simulink model "ANPC_BTB_precharge"  (Simulink 7.3)
settings: Solver=FixedStepDiscrete  StartTime=0.0  StopTime=5  FixedStep=10e-6  RelTol=1e-3
undefined symbols (not defined in the file or in its folder): C, Cd, Cf, Lg
libraries: powerlib x112, simulink x1
settings Model: Creator=wangkui02  LastModifiedBy=wangkui

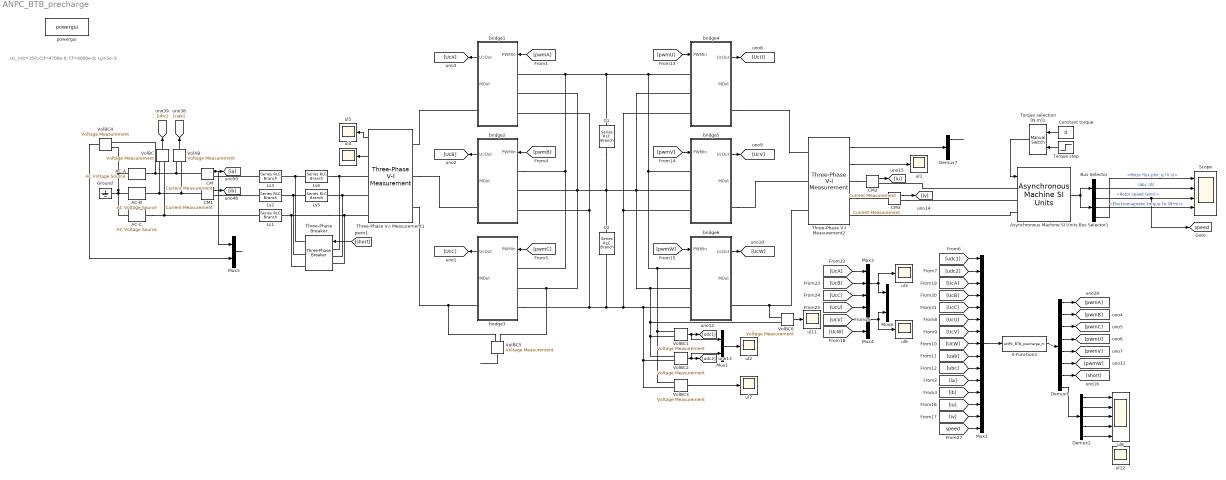
== system ANPC_BTB_precharge ==
  note: Uc_init=150;
      | Cd=4700e-6;
      | Cf=6600e-6;
      | Lg=5e-3;
  AC-A : powerlib/Electrical Sources/AC Voltage Source  DialogController=POWERSYS.PowerSysDialog  SystemSampleTime=-1  Amplitude=311  Phase=0  Frequency=50  SampleTime=0  Measurements=None
  AC-B : powerlib/Electrical Sources/AC Voltage Source  DialogController=POWERSYS.PowerSysDialog  SystemSampleTime=-1  Amplitude=311  Phase=-120  Frequency=50  SampleTime=0  Measurements=None
  AC-C : powerlib/Electrical Sources/AC Voltage Source  DialogController=POWERSYS.PowerSysDialog  SystemSampleTime=-1  Amplitude=311  Phase=120  Frequency=50  SampleTime=0  Measurements=None
  Asynchronous Machine SI Units : powerlib/Machines/Asynchronous Machine SI Units  DialogController=POWERSYS.PowerSysDialog  SystemSampleTime=-1  PresetModel=No  MechanicalLoad=Torque Tm  ShowDetailedParameters=on  RotorType=Squirrel-cage  ReferenceFrame=Stationary  NominalParameters=[2200 380 50]  Stator=[2.74 0.0138]  Rotor=[2.54 0.0138]  Lm=0.299  Mechanical=[0.0131 0.002985 2]  PolePairs=2  InitialConditions="[ 1,0   0,0,0   0,0,0 ]"  Units=SI  LoadFlowParameters=0  SimulateSaturation=off  Saturation=[14.03593122, 27.81365428, 53.79336849, 72.68890987, 97.98006896, 148.6815601, 215.7428561, 302.9841135, 428.7778367 ; 230, 322, 414, 460, 506, 552, 598, 644, 690]  TsPowergui=0  TsBlock=-1  IterativeModel=Forward Euler
  Bus Selector : BusSelector  OutputSignals=Stator measurements.Stator current is_a (A),Stator measurements.Stator current is_b (A),Stator measurements.Stator current is_c (A)  OutputAsBus=on
  Bus Selector1 : BusSelector  OutputSignals=Mechanical.Rotor speed (wm),Mechanical.Electromagnetic torque Te (N*m),Rotor measurements.Rotor flux phir_q (V s)
  C1 : powerlib/Elements/Series RLC Branch  DialogController=POWERSYS.PowerSysDialog  PhysicalDomain=powersysdomain  SubClassName=unknown  LeftPortType=p1  RightPortType=p1  LConnTagsString=__new0  RConnTagsString=__new0  BranchType=C  Resistance=1  Inductance=1e-3  SetiL0=off  InitialCurrent=0  Capacitance=Cd  Setx0=on  InitialVoltage=0  Measurements=None
  C2 : powerlib/Elements/Series RLC Branch  DialogController=POWERSYS.PowerSysDialog  PhysicalDomain=powersysdomain  SubClassName=unknown  LeftPortType=p1  RightPortType=p1  LConnTagsString=__new0  RConnTagsString=__new0  BranchType=C  Resistance=1  Inductance=1e-3  SetiL0=off  InitialCurrent=0  Capacitance=Cd  Setx0=on  InitialVoltage=0  Measurements=None
  CM{,1..3} (4 alike) : powerlib/Measurements/Current Measurement  DialogController=POWERSYS.PowerSysDialog  SystemSampleTime=-1  PhasorSimulation=off  OutputType=Complex  PSBequivalent=0
  Constant torque : Constant  Value=0  OutDataType=sfix(16)  OutScaling=2^0
  Demux1 : Demux  Outputs=[12 12 12 12 12 12 1 5]
  Demux2 : Demux  Outputs=5
  Demux7 : Demux  Outputs=3
  Ground : powerlib/Elements/Ground  DialogController=POWERSYS.PowerSysDialog  PhysicalDomain=powersysdomain  SubClassName=unknown  LeftPortType=p1  RightPortType=p1  LConnTagsString=a
  Ls1 : powerlib/Elements/Series RLC Branch  DialogController=POWERSYS.PowerSysDialog  PhysicalDomain=powersysdomain  SubClassName=unknown  LeftPortType=p1  RightPortType=p1  LConnTagsString=__new0  RConnTagsString=__new0  BranchType=L  Resistance=1  Inductance=Lg  SetiL0=off  InitialCurrent=0  Capacitance=C  Setx0=on  InitialVoltage=Uc  Measurements=Branch voltage and current
  Ls2 : powerlib/Elements/Series RLC Branch  DialogController=POWERSYS.PowerSysDialog  PhysicalDomain=powersysdomain  SubClassName=unknown  LeftPortType=p1  RightPortType=p1  LConnTagsString=__new0  RConnTagsString=__new0  BranchType=L  Resistance=1  Inductance=Lg  SetiL0=off  InitialCurrent=0  Capacitance=C  Setx0=on  InitialVoltage=Uc  Measurements=Branch voltage and current
  Ls3 : powerlib/Elements/Series RLC Branch  DialogController=POWERSYS.PowerSysDialog  PhysicalDomain=powersysdomain  SubClassName=unknown  LeftPortType=p1  RightPortType=p1  LConnTagsString=__new0  RConnTagsString=__new0  BranchType=L  Resistance=1  Inductance=Lg  SetiL0=off  InitialCurrent=0  Capacitance=C  Setx0=on  InitialVoltage=Uc  Measurements=Branch voltage and current
  Ls5 : powerlib/Elements/Series RLC Branch  DialogController=POWERSYS.PowerSysDialog  PhysicalDomain=powersysdomain  SubClassName=unknown  LeftPortType=p1  RightPortType=p1  LConnTagsString=__new0  RConnTagsString=__new0  BranchType=R  Resistance=20  Inductance=Lg  SetiL0=off  InitialCurrent=0  Capacitance=C  Setx0=on  InitialVoltage=Uc  Measurements=Branch voltage and current
  Ls6 : powerlib/Elements/Series RLC Branch  DialogController=POWERSYS.PowerSysDialog  PhysicalDomain=powersysdomain  SubClassName=unknown  LeftPortType=p1  RightPortType=p1  LConnTagsString=__new0  RConnTagsString=__new0  BranchType=R  Resistance=20  Inductance=Lg  SetiL0=off  InitialCurrent=0  Capacitance=C  Setx0=on  InitialVoltage=Uc  Measurements=Branch voltage and current
  Mux1 : Mux  Inputs=2
  Mux2 : Mux  Inputs=15
  Mux3 : Mux  Inputs=3
  Mux4 : Mux  Inputs=3
  Mux5 : Mux  Inputs=2
  Mux6 : Mux  Inputs=2
  S-Function2 : S-Function  FunctionName=ANPC_BTB_precharge_m  EnableBusSupport=off
  Scope : Scope  NumInputPorts=4
      settings: YMin=-1~-12.5~-10~-2.5  YMax=1~12.5~110~22.5  SaveName=ScopeData9  Decimation=20  SampleTime=5e-6
  Three-Phase V-I Measurement1 : powerlib/Measurements/Three-Phase V-I Measurement  DialogController=POWERSYS.PowerSysDialog  SystemSampleTime=-1  VoltageMeasurement=phase-to-phase  SetLabelV=off  LabelV=Vabc  Vpu=off  CurrentMeasurement=yes  SetLabelI=off  LabelI=Iabc  Ipu=off  Pbase=100e6  Vbase=500e3  OutputType=Complex  PhasorSimulation=off  PSBequivalent=0
  Three-Phase V-I Measurement2 : powerlib/Measurements/Three-Phase V-I Measurement  DialogController=POWERSYS.PowerSysDialog  SystemSampleTime=-1  VoltageMeasurement=phase-to-phase  SetLabelV=off  LabelV=Vabc  Vpu=off  CurrentMeasurement=yes  SetLabelI=off  LabelI=Iabc  Ipu=off  Pbase=100e6  Vbase=500e3  OutputType=Complex  PhasorSimulation=off  PSBequivalent=0
  Three-Phase Breaker : powerlib/Elements/Three-Phase Breaker  DialogController=POWERSYS.PowerSysDialog  SystemSampleTime=-1  InitialState=open  SwitchA=on  SwitchB=on  SwitchC=on  SwitchTimes="[4/60  10/60]"  External=on  BreakerResistance=0.001  SnubberResistance=1e6  SnubberCapacitance=inf  Measurements=None
  Torque selection (N.m)1 : simulink/Signal Routing/Manual Switch  SystemSampleTime=-1  sw=0  action=0  varsize=off
  Torque step : Step  Time=3.5  After=10  SampleTime=0
  VolAB : powerlib/Measurements/Voltage Measurement  DialogController=POWERSYS.PowerSysDialog  SystemSampleTime=-1  PhasorSimulation=off  OutputType=Complex  PSBequivalent=0
  VolBC{,1..6} (7 alike) : powerlib/Measurements/Voltage Measurement  DialogController=POWERSYS.PowerSysDialog  SystemSampleTime=-1  PhasorSimulation=off  OutputType=Complex  PSBequivalent=0
  bridge1 : Subsystem
  bridge2 : Subsystem
  bridge3 : Subsystem
  bridge4 : Subsystem
  bridge5 : Subsystem
  bridge6 : Subsystem
  powergui : powerlib/powergui  SystemSampleTime=-1  SimulationMode=Discrete  SampleTime=10e-6  frequency=60  SPID=off  DisableSnubberDevices=off  DisableRonSwitches=off  DisableVfSwitches=off  SwTol=0  Interpol=off  frequencyindice=0  echomessages=off  HookPort=off  DisplayEquations=off  FunctionMessages=off  EnableUseOfTLC=off  x0status=blocks  RestoreLinks=warning  Frange=[0:2:500]  Ylog=off  Xlog=on  ShowGrid=off  save=off  variable=ZData  ZoomFFT=on  StartTime=0.0  cycles=1  DisplayStyle=1  fundamental=60  FreqAxis=off  MaxFrequency=1000  frequencyindicesteady=1  RmsSteady=1  display=off  Ts=0  methode=off
  ul{1..7,11..12} (9 alike) : Scope
      ul1 settings: YMin=-4  YMax=6  DataFormat=Structure  MaxDataPoints=100000  Decimation=10
      ul11 settings: YMin=-350  YMax=350  SaveName=ScopeData11  DataFormat=Structure  MaxDataPoints=100000  Decimation=10
      ul12 settings: YMin=-2  YMax=4  SaveName=ScopeData12  DataFormat=Structure  MaxDataPoints=100000  Decimation=10
      ul2 settings: TimeRange=1  YMin=297.5  YMax=302.5  SaveName=ScopeData2  DataFormat=Structure  MaxDataPoints=100000  Decimation=10
      ul3 settings: YMin=149.3  YMax=150.7  DataFormat=Structure  MaxDataPoints=100000  Decimation=10
      ul4 settings: YMin=-11  YMax=11  SaveName=ScopeData3  DataFormat=Structure  MaxDataPoints=100000  Decimation=10
      ul5 settings: YMin=-0.0225  YMax=0.0225  SaveName=ScopeData4  DataFormat=Structure  MaxDataPoints=100000  Decimation=10
      ul6 settings: YMin=0  YMax=160  SaveName=ScopeData5  DataFormat=Structure  MaxDataPoints=100000  Decimation=10
      ul7 settings: YMin=599  YMax=601.4  SaveName=ScopeData6  DataFormat=Structure  MaxDataPoints=100000  Decimation=10
  ul8 : Scope  NumInputPorts=5
      settings: YMin=-15~-5~0~-1.25e-013~-4  YMax=40~30~350~1.25e-013~4  SaveName=ScopeData7  DataFormat=Structure  MaxDataPoints=100000
  tag scope: speed=global
  wires:
  VolAB/1 -> [uab]
  VolBC/1 -> [ubc]
  [pwmB] -> bridge2/1(PWMIn)
  [pwmC] -> bridge3/1(PWMIn)
  CM/1 -> [ia], Mux5/1
  CM1/1 -> [ib]
  [pwmU] -> bridge4/1(PWMIn)
  [pwmV] -> bridge5/1(PWMIn)
  [pwmW] -> bridge6/1(PWMIn)
  bridge4/1(UcOut) -> [UcU]
  bridge5/1(UcOut) -> [UcV]
  bridge6/1(UcOut) -> [UcW]
  [pwmA] -> bridge1/1(PWMIn)
  bridge3/1(UcOut) -> [UcC]
  bridge2/1(UcOut) -> [UcB]
  bridge1/1(UcOut) -> [UcA]
  Three-Phase V-I Measurement2/2 -> ul1/1
  Demux7/1 -> ?
  Three-Phase V-I Measurement2/1 -> Demux7/1
  CM2/1 -> [iu]
  CM3/1 -> [iv]
  VolBC2/1 -> [udc2], Mux1/2
  VolBC1/1 -> [udc1], Mux1/1
  Mux1/1 -> ul2/1
  VolBC3/1 -> ul7/1
  Three-Phase V-I Measurement1/1 -> ul5/1
  Three-Phase V-I Measurement1/2 -> ul4/1
  Mux5/1 -> ?
  VolBC4/1 -> Mux5/2
  Mux2/1 -> S-Function2/1
  S-Function2/1 -> Demux1/1
  Demux1/1 -> [pwmA]
  Demux1/2 -> [pwmB]
  Demux1/3 -> [pwmC]
  [udc1] -> Mux2/1
  [udc2] -> Mux2/2
  [UcA] -> Mux2/3
  [UcB] -> Mux2/4
  [UcC] -> Mux2/5
  [UcU] -> Mux2/6
  [UcV] -> Mux2/7
  [UcW] -> Mux2/8
  [uab] -> Mux2/9
  [ubc] -> Mux2/10
  [ia] -> Mux2/11
  [ib] -> Mux2/12
  [iu] -> Mux2/13
  [iv] -> Mux2/14
  Demux1/4 -> [pwmU]
  Demux1/5 -> [pwmV]
  Demux1/6 -> [pwmW]
  Demux2/3 -> ul8/3
  Demux2/1 -> ul8/1
  Demux2/2 -> ul8/2
  Demux2/4 -> ul8/4
  [speed] -> Mux2/15
  [UcA] -> Mux3/1
  [UcB] -> Mux3/2
  [UcC] -> Mux3/3
  [UcU] -> Mux4/1
  [UcV] -> Mux4/2
  [UcW] -> Mux4/3
  VolBC5/1 -> ?
  VolBC6/1 -> ul11/1
  Mux3/1 -> Mux6/1, ul3/1
  Mux4/1 -> Mux6/2, ul6/1
  Bus Selector1/1 -> Scope/3, [speed]  "<Rotor speed (wm)>"
  Bus Selector/1 -> Scope/2  "Iabc (A)"
  Bus Selector1/2 -> Scope/4  "<Electromagnetic torque Te (N*m)>"
  Asynchronous Machine SI Units/1 -> Bus Selector/1, Bus Selector1/1
  Torque selection (N.m)1/1 -> Asynchronous Machine SI Units/1
  Constant torque/1 -> Torque selection (N.m)1/1
  Torque step/1 -> Torque selection (N.m)1/2
  Bus Selector1/3 -> Scope/1  "<Rotor flux phir_q (V s)>"
  [short] -> Three-Phase Breaker/1
  Demux1/8 -> Demux2/1
  Demux1/7 -> [short]
  Demux2/5 -> ul8/5
  connections:
  AC-A/RConn1 -- VolAB/LConn1 -- CM/LConn1 -- VolBC4/LConn1
  AC-C/RConn1 -- Ls1/LConn1 -- VolBC/LConn2
  Ground/LConn1 -- AC-B/LConn1 -- AC-C/LConn1 -- AC-A/LConn1 -- VolBC4/LConn2
  Three-Phase V-I Measurement1/LConn1 -- bridge1/RConn1
  Three-Phase V-I Measurement1/LConn2 -- bridge2/RConn1
  Three-Phase V-I Measurement1/LConn3 -- bridge3/RConn1 -- VolBC5/LConn1
  CM1/RConn1 -- Ls2/LConn1
  Ls3/LConn1 -- CM/RConn1
  bridge6/LConn1 -- bridge3/LConn1 -- bridge2/LConn1 -- bridge1/LConn1 -- C1/LConn1 -- bridge4/LConn1 -- bridge5/LConn1 -- VolBC1/LConn1 -- VolBC3/LConn1
  bridge6/LConn3 -- bridge3/LConn3 -- bridge1/LConn3 -- bridge2/LConn3 -- C2/RConn1 -- bridge4/LConn3 -- bridge5/LConn3 -- VolBC2/LConn2 -- VolBC3/LConn2
  bridge4/RConn1 -- Three-Phase V-I Measurement2/LConn1
  bridge5/RConn1 -- Three-Phase V-I Measurement2/LConn2
  bridge6/RConn1 -- Three-Phase V-I Measurement2/LConn3 -- VolBC6/LConn1
  VolBC/LConn1 -- AC-B/RConn1 -- CM1/LConn1 -- VolAB/LConn2
  Three-Phase V-I Measurement2/RConn1 -- CM2/LConn1
  Three-Phase V-I Measurement2/RConn2 -- CM3/LConn1
  VolBC2/LConn1 -- VolBC1/LConn2 -- C2/LConn1 -- bridge2/LConn2 -- bridge1/LConn2 -- bridge3/LConn2 -- VolBC5/LConn2 -- C1/RConn1 -- bridge4/LConn2 -- bridge5/LConn2 -- bridge6/LConn2 -- VolBC6/LConn2
  CM3/RConn1 -- Asynchronous Machine SI Units/LConn2
  Three-Phase V-I Measurement2/RConn3 -- Asynchronous Machine SI Units/LConn3
  Asynchronous Machine SI Units/LConn1 -- CM2/RConn1
  Ls6/LConn1 -- Ls3/RConn1 -- Three-Phase Breaker/RConn1
  Ls5/LConn1 -- Ls2/RConn1 -- Three-Phase Breaker/RConn2
  Ls6/RConn1 -- Three-Phase V-I Measurement1/RConn1 -- Three-Phase Breaker/LConn1
  Ls5/RConn1 -- Three-Phase V-I Measurement1/RConn2 -- Three-Phase Breaker/LConn2
  Ls1/RConn1 -- Three-Phase Breaker/RConn3 -- Three-Phase V-I Measurement1/RConn3 -- Three-Phase Breaker/LConn3

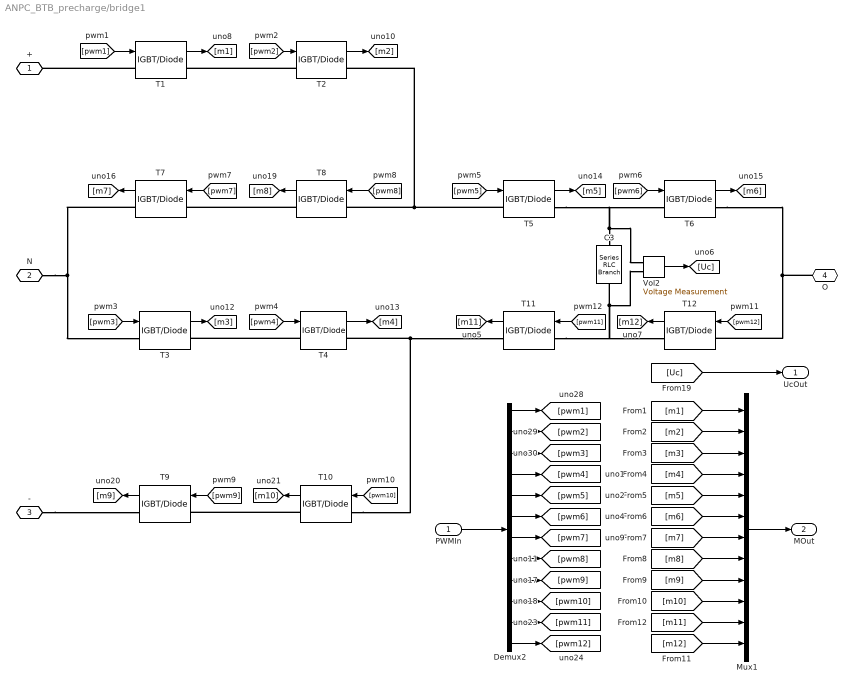
== system ANPC_BTB_precharge/bridge1 ==
  PWMIn : Inport
  C3 : powerlib/Elements/Series RLC Branch  DialogController=POWERSYS.PowerSysDialog  PhysicalDomain=powersysdomain  SubClassName=unknown  LeftPortType=p1  RightPortType=p1  LConnTagsString=__new0  RConnTagsString=__new0  BranchType=C  Resistance=1  Inductance=1e-3  SetiL0=off  InitialCurrent=0  Capacitance=Cf  Setx0=on  InitialVoltage=0  Measurements=None
  Demux2 : Demux  Outputs=12
  Mux1 : Mux  Inputs=12
  T{1..12} (12 alike) : powerlib/Power Electronics/IGBT//Diode  DialogController=POWERSYS.PowerSysDialog  SystemSampleTime=-1  Ron=1e-3  Rs=1e5  Cs=inf  Measurements=on
  Vol2 : powerlib/Measurements/Voltage Measurement  DialogController=POWERSYS.PowerSysDialog  SystemSampleTime=-1  PhasorSimulation=off  OutputType=Complex  PSBequivalent=0
  + : PMIOPort  Port=1  Side=Left
  N : PMIOPort  Port=2  Side=Left
  - : PMIOPort  Port=3  Side=Left
  O : PMIOPort  Port=4  Side=Right
  UcOut : Outport  OutDataType=fixdt(1, 16)  OutScaling=2^0
  MOut : Outport  Port=2  OutDataType=fixdt(1, 16)  OutScaling=2^0
  wires:
  T1/1 -> [m1]
  [pwm10] -> T10/1
  T10/1 -> [m10]
  [pwm3] -> T3/1
  T3/1 -> [m3]
  [pwm4] -> T4/1
  T4/1 -> [m4]
  [pwm5] -> T5/1
  T5/1 -> [m5]
  [pwm2] -> T2/1
  T2/1 -> [m2]
  [pwm6] -> T6/1
  T6/1 -> [m6]
  [pwm7] -> T7/1
  [pwm8] -> T8/1
  T8/1 -> [m8]
  [pwm9] -> T9/1
  T9/1 -> [m9]
  PWMIn/1 -> Demux2/1
  Demux2/1 -> [pwm1]
  Demux2/2 -> [pwm2]
  Demux2/3 -> [pwm3]
  Demux2/4 -> [pwm4]
  Demux2/5 -> [pwm5]
  Demux2/6 -> [pwm6]
  Demux2/7 -> [pwm7]
  Demux2/8 -> [pwm8]
  Demux2/9 -> [pwm9]
  Demux2/10 -> [pwm10]
  [pwm1] -> T1/1
  T7/1 -> [m7]
  [m1] -> Mux1/1
  [m2] -> Mux1/2
  [m3] -> Mux1/3
  [m4] -> Mux1/4
  [m5] -> Mux1/5
  [m6] -> Mux1/6
  [m7] -> Mux1/7
  [m8] -> Mux1/8
  [m9] -> Mux1/9
  [m10] -> Mux1/10
  Mux1/1 -> MOut/1
  [pwm12] -> T12/1
  T12/1 -> [m12]
  [pwm11] -> T11/1
  T11/1 -> [m11]
  Vol2/1 -> [Uc]
  Demux2/11 -> [pwm11]
  Demux2/12 -> [pwm12]
  [m11] -> Mux1/11
  [m12] -> Mux1/12
  [Uc] -> UcOut/1
  connections:
  T2/LConn1 -- T1/RConn1
  T8/RConn1 -- T7/LConn1
  T1/LConn1 -- +/RConn1
  T7/RConn1 -- T3/LConn1 -- N/RConn1
  -/RConn1 -- T9/RConn1
  T4/LConn1 -- T3/RConn1
  T10/RConn1 -- T9/LConn1
  T11/LConn1 -- T12/RConn1 -- C3/RConn1 -- Vol2/LConn2
  T5/RConn1 -- T6/LConn1 -- C3/LConn1 -- Vol2/LConn1
  T5/LConn1 -- T2/RConn1 -- T8/LConn1
  T10/LConn1 -- T4/RConn1 -- T11/RConn1
  T6/RConn1 -- T12/LConn1 -- O/RConn1

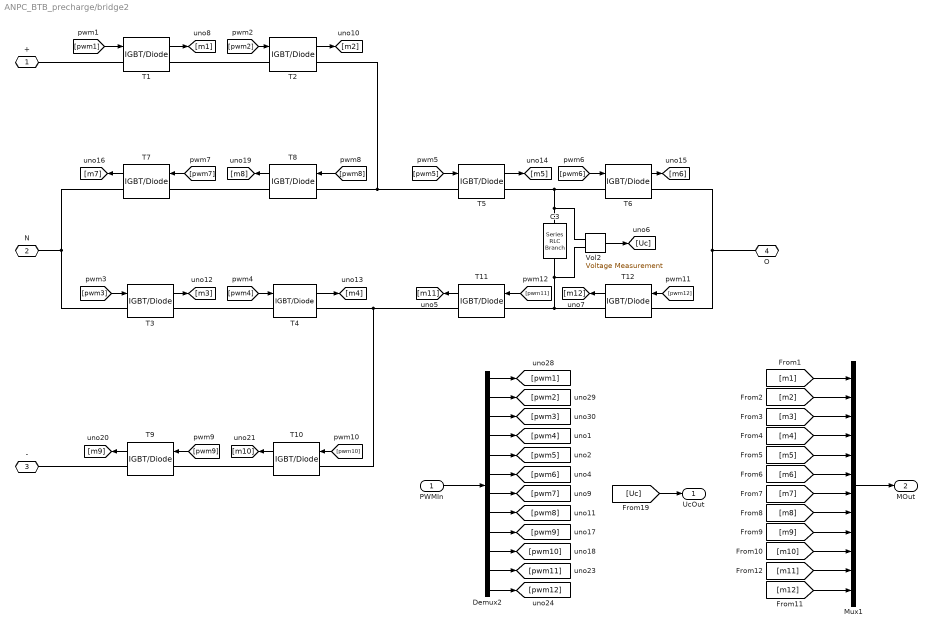
== system ANPC_BTB_precharge/bridge2 ==
  PWMIn : Inport
  C3 : powerlib/Elements/Series RLC Branch  DialogController=POWERSYS.PowerSysDialog  PhysicalDomain=powersysdomain  SubClassName=unknown  LeftPortType=p1  RightPortType=p1  LConnTagsString=__new0  RConnTagsString=__new0  BranchType=C  Resistance=1  Inductance=1e-3  SetiL0=off  InitialCurrent=0  Capacitance=Cf  Setx0=on  InitialVoltage=0  Measurements=None
  Demux2 : Demux  Outputs=12
  Mux1 : Mux  Inputs=12
  T{1..12} (12 alike) : powerlib/Power Electronics/IGBT//Diode  DialogController=POWERSYS.PowerSysDialog  SystemSampleTime=-1  Ron=1e-3  Rs=1e5  Cs=inf  Measurements=on
  Vol2 : powerlib/Measurements/Voltage Measurement  DialogController=POWERSYS.PowerSysDialog  SystemSampleTime=-1  PhasorSimulation=off  OutputType=Complex  PSBequivalent=0
  + : PMIOPort  Port=1  Side=Left
  N : PMIOPort  Port=2  Side=Left
  - : PMIOPort  Port=3  Side=Left
  O : PMIOPort  Port=4  Side=Right
  UcOut : Outport  OutDataType=fixdt(1, 16)  OutScaling=2^0
  MOut : Outport  Port=2  OutDataType=fixdt(1, 16)  OutScaling=2^0
  wires:
  T1/1 -> [m1]
  [pwm10] -> T10/1
  T10/1 -> [m10]
  [pwm3] -> T3/1
  T3/1 -> [m3]
  [pwm4] -> T4/1
  T4/1 -> [m4]
  [pwm5] -> T5/1
  T5/1 -> [m5]
  [pwm2] -> T2/1
  T2/1 -> [m2]
  [pwm6] -> T6/1
  T6/1 -> [m6]
  [pwm7] -> T7/1
  [pwm8] -> T8/1
  T8/1 -> [m8]
  [pwm9] -> T9/1
  T9/1 -> [m9]
  PWMIn/1 -> Demux2/1
  Demux2/1 -> [pwm1]
  Demux2/2 -> [pwm2]
  Demux2/3 -> [pwm3]
  Demux2/4 -> [pwm4]
  Demux2/5 -> [pwm5]
  Demux2/6 -> [pwm6]
  Demux2/7 -> [pwm7]
  Demux2/8 -> [pwm8]
  Demux2/9 -> [pwm9]
  Demux2/10 -> [pwm10]
  [pwm1] -> T1/1
  T7/1 -> [m7]
  [m1] -> Mux1/1
  [m2] -> Mux1/2
  [m3] -> Mux1/3
  [m4] -> Mux1/4
  [m5] -> Mux1/5
  [m6] -> Mux1/6
  [m7] -> Mux1/7
  [m8] -> Mux1/8
  [m9] -> Mux1/9
  [m10] -> Mux1/10
  Mux1/1 -> MOut/1
  [pwm12] -> T12/1
  T12/1 -> [m12]
  [pwm11] -> T11/1
  T11/1 -> [m11]
  Vol2/1 -> [Uc]
  Demux2/11 -> [pwm11]
  Demux2/12 -> [pwm12]
  [m11] -> Mux1/11
  [m12] -> Mux1/12
  [Uc] -> UcOut/1
  connections:
  T2/LConn1 -- T1/RConn1
  T8/RConn1 -- T7/LConn1
  T1/LConn1 -- +/RConn1
  T7/RConn1 -- T3/LConn1 -- N/RConn1
  -/RConn1 -- T9/RConn1
  T4/LConn1 -- T3/RConn1
  T10/RConn1 -- T9/LConn1
  T11/LConn1 -- T12/RConn1 -- C3/RConn1 -- Vol2/LConn2
  T5/RConn1 -- T6/LConn1 -- C3/LConn1 -- Vol2/LConn1
  T5/LConn1 -- T2/RConn1 -- T8/LConn1
  T10/LConn1 -- T4/RConn1 -- T11/RConn1
  T6/RConn1 -- T12/LConn1 -- O/RConn1

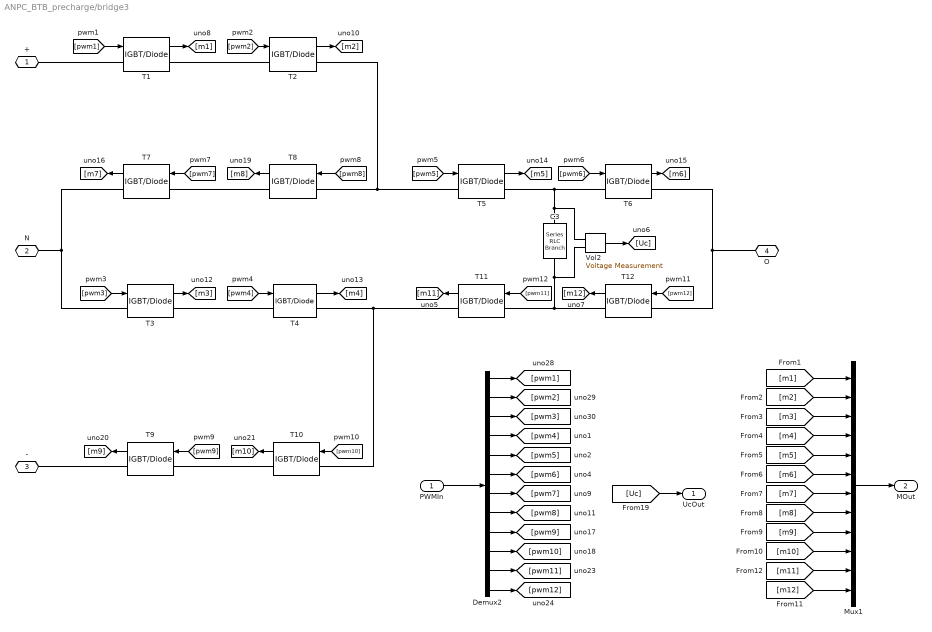
== system ANPC_BTB_precharge/bridge3 ==
  PWMIn : Inport
  C3 : powerlib/Elements/Series RLC Branch  DialogController=POWERSYS.PowerSysDialog  PhysicalDomain=powersysdomain  SubClassName=unknown  LeftPortType=p1  RightPortType=p1  LConnTagsString=__new0  RConnTagsString=__new0  BranchType=C  Resistance=1  Inductance=1e-3  SetiL0=off  InitialCurrent=0  Capacitance=Cf  Setx0=on  InitialVoltage=0  Measurements=None
  Demux2 : Demux  Outputs=12
  Mux1 : Mux  Inputs=12
  T{1..12} (12 alike) : powerlib/Power Electronics/IGBT//Diode  DialogController=POWERSYS.PowerSysDialog  SystemSampleTime=-1  Ron=1e-3  Rs=1e5  Cs=inf  Measurements=on
  Vol2 : powerlib/Measurements/Voltage Measurement  DialogController=POWERSYS.PowerSysDialog  SystemSampleTime=-1  PhasorSimulation=off  OutputType=Complex  PSBequivalent=0
  + : PMIOPort  Port=1  Side=Left
  N : PMIOPort  Port=2  Side=Left
  - : PMIOPort  Port=3  Side=Left
  O : PMIOPort  Port=4  Side=Right
  UcOut : Outport  OutDataType=fixdt(1, 16)  OutScaling=2^0
  MOut : Outport  Port=2  OutDataType=fixdt(1, 16)  OutScaling=2^0
  wires:
  T1/1 -> [m1]
  [pwm10] -> T10/1
  T10/1 -> [m10]
  [pwm3] -> T3/1
  T3/1 -> [m3]
  [pwm4] -> T4/1
  T4/1 -> [m4]
  [pwm5] -> T5/1
  T5/1 -> [m5]
  [pwm2] -> T2/1
  T2/1 -> [m2]
  [pwm6] -> T6/1
  T6/1 -> [m6]
  [pwm7] -> T7/1
  [pwm8] -> T8/1
  T8/1 -> [m8]
  [pwm9] -> T9/1
  T9/1 -> [m9]
  PWMIn/1 -> Demux2/1
  Demux2/1 -> [pwm1]
  Demux2/2 -> [pwm2]
  Demux2/3 -> [pwm3]
  Demux2/4 -> [pwm4]
  Demux2/5 -> [pwm5]
  Demux2/6 -> [pwm6]
  Demux2/7 -> [pwm7]
  Demux2/8 -> [pwm8]
  Demux2/9 -> [pwm9]
  Demux2/10 -> [pwm10]
  [pwm1] -> T1/1
  T7/1 -> [m7]
  [m1] -> Mux1/1
  [m2] -> Mux1/2
  [m3] -> Mux1/3
  [m4] -> Mux1/4
  [m5] -> Mux1/5
  [m6] -> Mux1/6
  [m7] -> Mux1/7
  [m8] -> Mux1/8
  [m9] -> Mux1/9
  [m10] -> Mux1/10
  Mux1/1 -> MOut/1
  [pwm12] -> T12/1
  T12/1 -> [m12]
  [pwm11] -> T11/1
  T11/1 -> [m11]
  Vol2/1 -> [Uc]
  Demux2/11 -> [pwm11]
  Demux2/12 -> [pwm12]
  [m11] -> Mux1/11
  [m12] -> Mux1/12
  [Uc] -> UcOut/1
  connections:
  T2/LConn1 -- T1/RConn1
  T8/RConn1 -- T7/LConn1
  T1/LConn1 -- +/RConn1
  T7/RConn1 -- T3/LConn1 -- N/RConn1
  -/RConn1 -- T9/RConn1
  T4/LConn1 -- T3/RConn1
  T10/RConn1 -- T9/LConn1
  T11/LConn1 -- T12/RConn1 -- C3/RConn1 -- Vol2/LConn2
  T5/RConn1 -- T6/LConn1 -- C3/LConn1 -- Vol2/LConn1
  T5/LConn1 -- T2/RConn1 -- T8/LConn1
  T10/LConn1 -- T4/RConn1 -- T11/RConn1
  T6/RConn1 -- T12/LConn1 -- O/RConn1

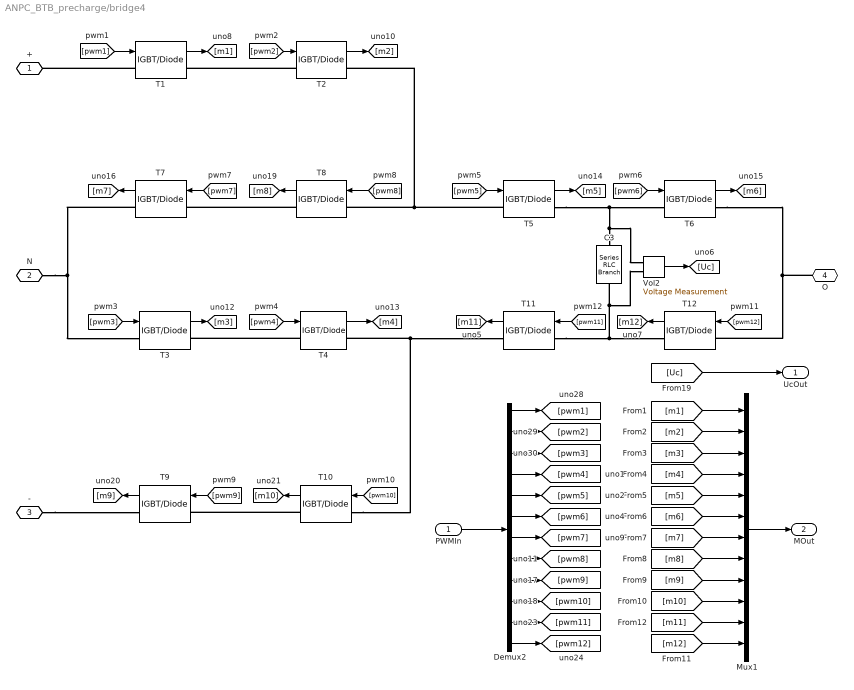
== system ANPC_BTB_precharge/bridge4 ==
  PWMIn : Inport
  C3 : powerlib/Elements/Series RLC Branch  DialogController=POWERSYS.PowerSysDialog  PhysicalDomain=powersysdomain  SubClassName=unknown  LeftPortType=p1  RightPortType=p1  LConnTagsString=__new0  RConnTagsString=__new0  BranchType=C  Resistance=1  Inductance=1e-3  SetiL0=off  InitialCurrent=0  Capacitance=Cf  Setx0=on  InitialVoltage=0  Measurements=None
  Demux2 : Demux  Outputs=12
  Mux1 : Mux  Inputs=12
  T{1..12} (12 alike) : powerlib/Power Electronics/IGBT//Diode  DialogController=POWERSYS.PowerSysDialog  SystemSampleTime=-1  Ron=1e-3  Rs=1e5  Cs=inf  Measurements=on
  Vol2 : powerlib/Measurements/Voltage Measurement  DialogController=POWERSYS.PowerSysDialog  SystemSampleTime=-1  PhasorSimulation=off  OutputType=Complex  PSBequivalent=0
  + : PMIOPort  Port=1  Side=Left
  N : PMIOPort  Port=2  Side=Left
  - : PMIOPort  Port=3  Side=Left
  O : PMIOPort  Port=4  Side=Right
  UcOut : Outport  OutDataType=fixdt(1, 16)  OutScaling=2^0
  MOut : Outport  Port=2  OutDataType=fixdt(1, 16)  OutScaling=2^0
  wires:
  T1/1 -> [m1]
  [pwm10] -> T10/1
  T10/1 -> [m10]
  [pwm3] -> T3/1
  T3/1 -> [m3]
  [pwm4] -> T4/1
  T4/1 -> [m4]
  [pwm5] -> T5/1
  T5/1 -> [m5]
  [pwm2] -> T2/1
  T2/1 -> [m2]
  [pwm6] -> T6/1
  T6/1 -> [m6]
  [pwm7] -> T7/1
  [pwm8] -> T8/1
  T8/1 -> [m8]
  [pwm9] -> T9/1
  T9/1 -> [m9]
  Demux2/1 -> [pwm1]
  Demux2/2 -> [pwm2]
  Demux2/3 -> [pwm3]
  Demux2/4 -> [pwm4]
  Demux2/5 -> [pwm5]
  Demux2/6 -> [pwm6]
  Demux2/7 -> [pwm7]
  Demux2/8 -> [pwm8]
  Demux2/9 -> [pwm9]
  Demux2/10 -> [pwm10]
  [pwm1] -> T1/1
  T7/1 -> [m7]
  [m1] -> Mux1/1
  [m2] -> Mux1/2
  [m3] -> Mux1/3
  [m4] -> Mux1/4
  [m5] -> Mux1/5
  [m6] -> Mux1/6
  [m7] -> Mux1/7
  [m8] -> Mux1/8
  [m9] -> Mux1/9
  [m10] -> Mux1/10
  [pwm12] -> T12/1
  T12/1 -> [m12]
  [pwm11] -> T11/1
  T11/1 -> [m11]
  Vol2/1 -> [Uc]
  Demux2/11 -> [pwm11]
  Demux2/12 -> [pwm12]
  [m11] -> Mux1/11
  [m12] -> Mux1/12
  [Uc] -> UcOut/1
  Mux1/1 -> MOut/1
  PWMIn/1 -> Demux2/1
  connections:
  T2/LConn1 -- T1/RConn1
  T8/RConn1 -- T7/LConn1
  T1/LConn1 -- +/RConn1
  T7/RConn1 -- T3/LConn1 -- N/RConn1
  -/RConn1 -- T9/RConn1
  T4/LConn1 -- T3/RConn1
  T10/RConn1 -- T9/LConn1
  T11/LConn1 -- T12/RConn1 -- C3/RConn1 -- Vol2/LConn2
  T5/RConn1 -- T6/LConn1 -- C3/LConn1 -- Vol2/LConn1
  T5/LConn1 -- T2/RConn1 -- T8/LConn1
  T10/LConn1 -- T4/RConn1 -- T11/RConn1
  T6/RConn1 -- T12/LConn1 -- O/RConn1

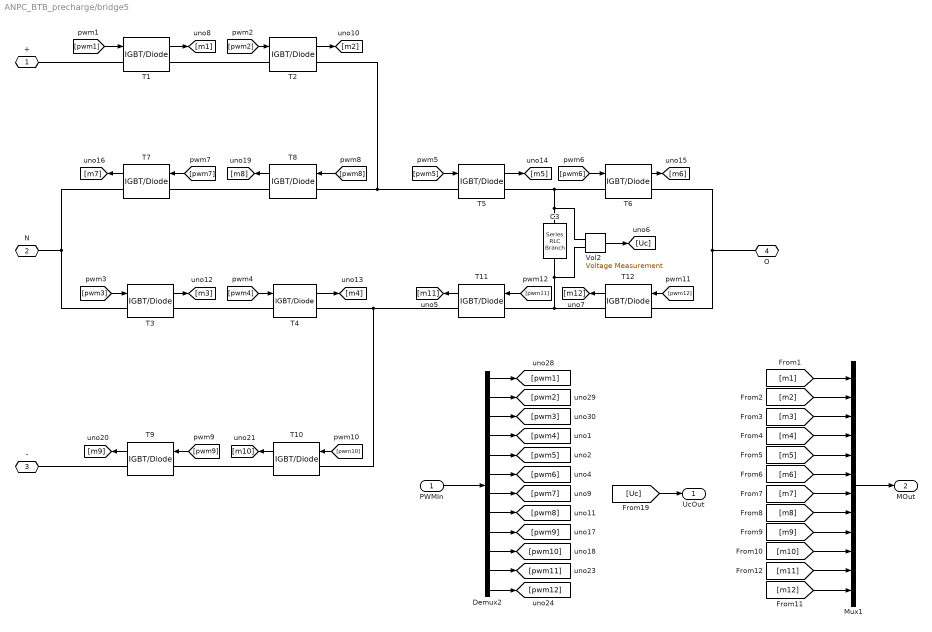
== system ANPC_BTB_precharge/bridge5 ==
  PWMIn : Inport
  C3 : powerlib/Elements/Series RLC Branch  DialogController=POWERSYS.PowerSysDialog  PhysicalDomain=powersysdomain  SubClassName=unknown  LeftPortType=p1  RightPortType=p1  LConnTagsString=__new0  RConnTagsString=__new0  BranchType=C  Resistance=1  Inductance=1e-3  SetiL0=off  InitialCurrent=0  Capacitance=Cf  Setx0=on  InitialVoltage=0  Measurements=None
  Demux2 : Demux  Outputs=12
  Mux1 : Mux  Inputs=12
  T{1..12} (12 alike) : powerlib/Power Electronics/IGBT//Diode  DialogController=POWERSYS.PowerSysDialog  SystemSampleTime=-1  Ron=1e-3  Rs=1e5  Cs=inf  Measurements=on
  Vol2 : powerlib/Measurements/Voltage Measurement  DialogController=POWERSYS.PowerSysDialog  SystemSampleTime=-1  PhasorSimulation=off  OutputType=Complex  PSBequivalent=0
  + : PMIOPort  Port=1  Side=Left
  N : PMIOPort  Port=2  Side=Left
  - : PMIOPort  Port=3  Side=Left
  O : PMIOPort  Port=4  Side=Right
  UcOut : Outport  OutDataType=fixdt(1, 16)  OutScaling=2^0
  MOut : Outport  Port=2  OutDataType=fixdt(1, 16)  OutScaling=2^0
  wires:
  T1/1 -> [m1]
  [pwm10] -> T10/1
  T10/1 -> [m10]
  [pwm3] -> T3/1
  T3/1 -> [m3]
  [pwm4] -> T4/1
  T4/1 -> [m4]
  [pwm5] -> T5/1
  T5/1 -> [m5]
  [pwm2] -> T2/1
  T2/1 -> [m2]
  [pwm6] -> T6/1
  T6/1 -> [m6]
  [pwm7] -> T7/1
  [pwm8] -> T8/1
  T8/1 -> [m8]
  [pwm9] -> T9/1
  T9/1 -> [m9]
  PWMIn/1 -> Demux2/1
  Demux2/1 -> [pwm1]
  Demux2/2 -> [pwm2]
  Demux2/3 -> [pwm3]
  Demux2/4 -> [pwm4]
  Demux2/5 -> [pwm5]
  Demux2/6 -> [pwm6]
  Demux2/7 -> [pwm7]
  Demux2/8 -> [pwm8]
  Demux2/9 -> [pwm9]
  Demux2/10 -> [pwm10]
  [pwm1] -> T1/1
  T7/1 -> [m7]
  [m1] -> Mux1/1
  [m2] -> Mux1/2
  [m3] -> Mux1/3
  [m4] -> Mux1/4
  [m5] -> Mux1/5
  [m6] -> Mux1/6
  [m7] -> Mux1/7
  [m8] -> Mux1/8
  [m9] -> Mux1/9
  [m10] -> Mux1/10
  Mux1/1 -> MOut/1
  [pwm12] -> T12/1
  T12/1 -> [m12]
  [pwm11] -> T11/1
  T11/1 -> [m11]
  Vol2/1 -> [Uc]
  Demux2/11 -> [pwm11]
  Demux2/12 -> [pwm12]
  [m11] -> Mux1/11
  [m12] -> Mux1/12
  [Uc] -> UcOut/1
  connections:
  T2/LConn1 -- T1/RConn1
  T8/RConn1 -- T7/LConn1
  T1/LConn1 -- +/RConn1
  T7/RConn1 -- T3/LConn1 -- N/RConn1
  -/RConn1 -- T9/RConn1
  T4/LConn1 -- T3/RConn1
  T10/RConn1 -- T9/LConn1
  T11/LConn1 -- T12/RConn1 -- C3/RConn1 -- Vol2/LConn2
  T5/RConn1 -- T6/LConn1 -- C3/LConn1 -- Vol2/LConn1
  T5/LConn1 -- T2/RConn1 -- T8/LConn1
  T10/LConn1 -- T4/RConn1 -- T11/RConn1
  T6/RConn1 -- T12/LConn1 -- O/RConn1

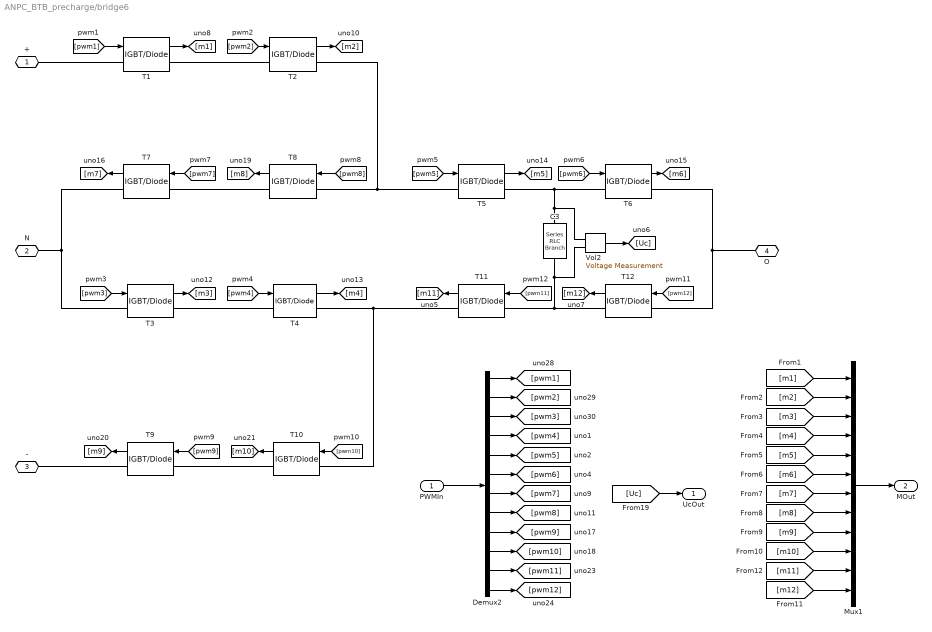
== system ANPC_BTB_precharge/bridge6 ==
  PWMIn : Inport
  C3 : powerlib/Elements/Series RLC Branch  DialogController=POWERSYS.PowerSysDialog  PhysicalDomain=powersysdomain  SubClassName=unknown  LeftPortType=p1  RightPortType=p1  LConnTagsString=__new0  RConnTagsString=__new0  BranchType=C  Resistance=1  Inductance=1e-3  SetiL0=off  InitialCurrent=0  Capacitance=Cf  Setx0=on  InitialVoltage=0  Measurements=None
  Demux2 : Demux  Outputs=12
  Mux1 : Mux  Inputs=12
  T{1..12} (12 alike) : powerlib/Power Electronics/IGBT//Diode  DialogController=POWERSYS.PowerSysDialog  SystemSampleTime=-1  Ron=1e-3  Rs=1e5  Cs=inf  Measurements=on
  Vol2 : powerlib/Measurements/Voltage Measurement  DialogController=POWERSYS.PowerSysDialog  SystemSampleTime=-1  PhasorSimulation=off  OutputType=Complex  PSBequivalent=0
  + : PMIOPort  Port=1  Side=Left
  N : PMIOPort  Port=2  Side=Left
  - : PMIOPort  Port=3  Side=Left
  O : PMIOPort  Port=4  Side=Right
  UcOut : Outport  OutDataType=fixdt(1, 16)  OutScaling=2^0
  MOut : Outport  Port=2  OutDataType=fixdt(1, 16)  OutScaling=2^0
  wires:
  T1/1 -> [m1]
  [pwm10] -> T10/1
  T10/1 -> [m10]
  [pwm3] -> T3/1
  T3/1 -> [m3]
  [pwm4] -> T4/1
  T4/1 -> [m4]
  [pwm5] -> T5/1
  T5/1 -> [m5]
  [pwm2] -> T2/1
  T2/1 -> [m2]
  [pwm6] -> T6/1
  T6/1 -> [m6]
  [pwm7] -> T7/1
  [pwm8] -> T8/1
  T8/1 -> [m8]
  [pwm9] -> T9/1
  T9/1 -> [m9]
  PWMIn/1 -> Demux2/1
  Demux2/1 -> [pwm1]
  Demux2/2 -> [pwm2]
  Demux2/3 -> [pwm3]
  Demux2/4 -> [pwm4]
  Demux2/5 -> [pwm5]
  Demux2/6 -> [pwm6]
  Demux2/7 -> [pwm7]
  Demux2/8 -> [pwm8]
  Demux2/9 -> [pwm9]
  Demux2/10 -> [pwm10]
  [pwm1] -> T1/1
  T7/1 -> [m7]
  [m1] -> Mux1/1
  [m2] -> Mux1/2
  [m3] -> Mux1/3
  [m4] -> Mux1/4
  [m5] -> Mux1/5
  [m6] -> Mux1/6
  [m7] -> Mux1/7
  [m8] -> Mux1/8
  [m9] -> Mux1/9
  [m10] -> Mux1/10
  Mux1/1 -> MOut/1
  [pwm12] -> T12/1
  T12/1 -> [m12]
  [pwm11] -> T11/1
  T11/1 -> [m11]
  Vol2/1 -> [Uc]
  Demux2/11 -> [pwm11]
  Demux2/12 -> [pwm12]
  [m11] -> Mux1/11
  [m12] -> Mux1/12
  [Uc] -> UcOut/1
  connections:
  T2/LConn1 -- T1/RConn1
  T8/RConn1 -- T7/LConn1
  T1/LConn1 -- +/RConn1
  T7/RConn1 -- T3/LConn1 -- N/RConn1
  -/RConn1 -- T9/RConn1
  T4/LConn1 -- T3/RConn1
  T10/RConn1 -- T9/LConn1
  T11/LConn1 -- T12/RConn1 -- C3/RConn1 -- Vol2/LConn2
  T5/RConn1 -- T6/LConn1 -- C3/LConn1 -- Vol2/LConn1
  T5/LConn1 -- T2/RConn1 -- T8/LConn1
  T10/LConn1 -- T4/RConn1 -- T11/RConn1
  T6/RConn1 -- T12/LConn1 -- O/RConn1
